simulink model "Drive_My_RRS"  (R2023b)
settings: Solver=VariableStepAuto  StartTime=0.0  StopTime=10.0  RelTol=1e-3
undefined symbols (not defined in the file or in its folder): X, Y, Z
libraries: sm_lib x48, nesl_utility x7, robotcorelib x1, robotmaniplib x1
(part 1 of 2)
settings Model: Creator=anthe  LastModifiedBy=anthe

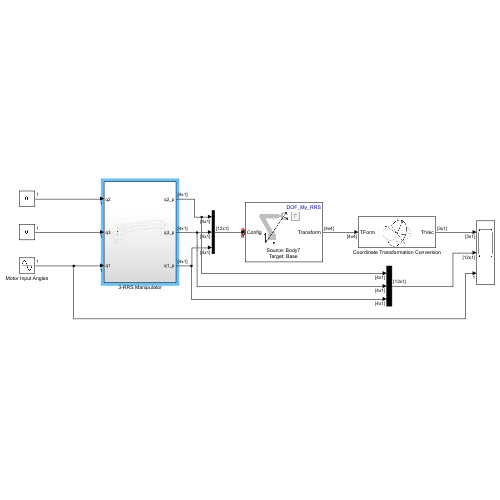
[thumbnail: Simulink's stored preview of the top-level diagram]
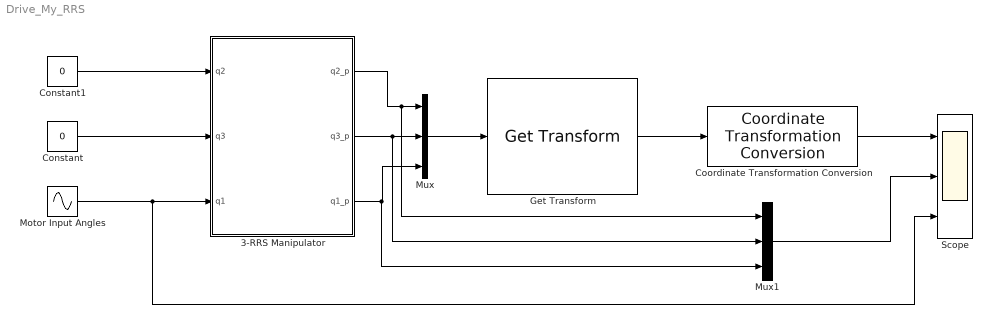
== system Drive_My_RRS ==
  3-RRS Manipulator : Subsystem
  Constant : Constant  Value=0
  Constant1 : Constant  Value=0
  Coordinate Transformation Conversion : robotcorelib/Coordinate Transformation Conversion  InputRepresentation=Homogeneous Transformation  InputEulerSequence=ZYX  ShowTrVecInputPort=on  OutputRepresentation=Translation Vector  OutputEulerSequence=ZYX  ShowTrVecOutputPort=on  SimulateUsing=Interpreted execution
  Get Transform : robotmaniplib/Get Transform  RigidBodyTree=DOF_My_RRS  SourceBody=Body7  TargetBody=Base  SimulateUsing=Interpreted execution
  Motor Input Angles : Sin  Amplitude=0.5  SampleTime=0
  Mux : Mux  Inputs=3
  Mux1 : Mux  Inputs=3
  Scope : Scope  NumInputPorts=3
  wires:
  Motor Input Angles/1 -> Scope/3, 3-RRS Manipulator/3(q1)
  Constant/1 -> 3-RRS Manipulator/2(q3)
  Constant1/1 -> 3-RRS Manipulator/1(q2)
  3-RRS Manipulator/3(q1_p) -> Mux1/3, Mux/3
  3-RRS Manipulator/2(q3_p) -> Mux1/2, Mux/2
  3-RRS Manipulator/1(q2_p) -> Mux1/1, Mux/1
  Mux/1 -> Get Transform/1
  Get Transform/1 -> Coordinate Transformation Conversion/1
  Coordinate Transformation Conversion/1 -> Scope/1
  Mux1/1 -> Scope/2
